simulink model "EcoSIM3_P2_C2"  (R2014b)
settings: Solver=ode1  SolverMode=SingleTasking  StartTime=0.0  StopTime=inf  FixedStep=0.01  RelTol=1e-3
PostLoadFcn:
  | %, if any(exist('dsrtsu_mdlpostloadfcn', 'file') == [2, 3, 6]), try dsrtsu_mdlpostloadfcn('Execute', bdroot); catch fprintf('Error in PostLoadFcn (dsrtsu_mdlpostloadfcn) for model "%s":\n %s\n', bdroot, lasterr); end, end,
InitFcn:
  | tic
  | %Startup_EcoSIM
undefined symbols (not defined in the file or in its folder): canChannel, Controls, DriveCycles, Driver, EM_EFF_MAP, EM_PwrLoss_MAP, EngPwr, EngSpd, EngTrq, Glbl, Plants, Power, Torque, Veh_Dynamics
libraries: canmsglib x100, canlib x87, fl_lib x78, simulink x59, nesl_utility x40, sdl_lib x17, dspsigops x5, dspswit3 x3, dspstat3 x2, commnoisgen2 x1, dspfdesign x1
(part 11 of 15)

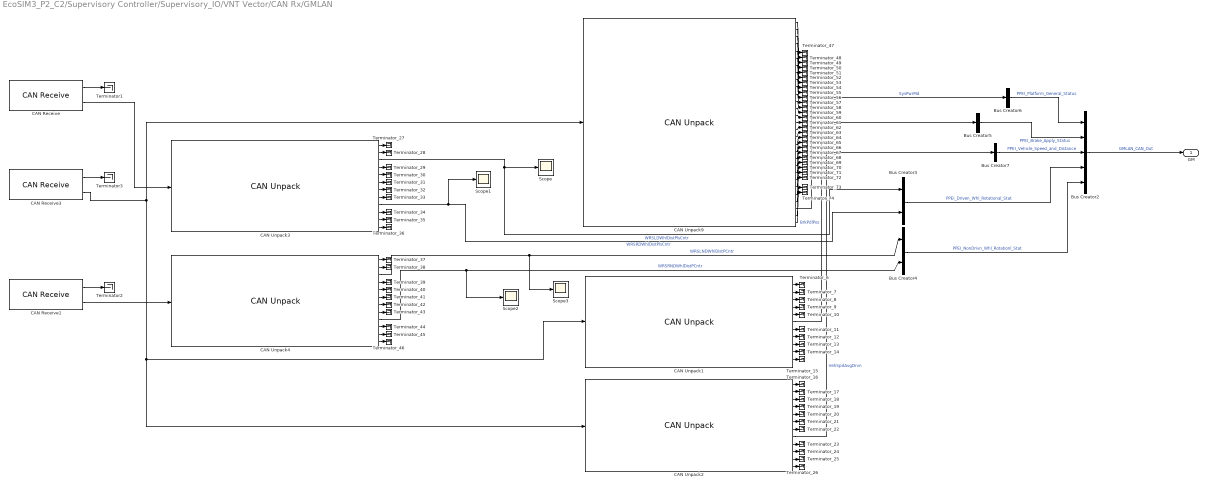
== system EcoSIM3_P2_C2/Supervisory Controller/Supervisory_IO/VNT Vector/CAN Rx/GMLAN ==
  Bus Creator2 : BusCreator  Inputs=5
  Bus Creator3 : BusCreator  Inputs=2
  Bus Creator4 : BusCreator  Inputs=2
  Bus Creator5 : BusCreator  Inputs=1
  Bus Creator6 : BusCreator  Inputs=1
  Bus Creator7 : BusCreator  Inputs=1
  CAN Receive : canlib/CAN Receive  BlockHandle=34350.0007  DeviceMenu=Vector Virtual 1 (Channel 1)  Device=Vector Virtual 1 (Channel 1)  ObjConstructor=canChannel('Vector', 'Virtual 1', 1)  EnableStandardIDsFilter=off  StandardIDs=193  EnableExtendedIDsFilter=off  ExtendedIDs=0  SampleTime=0.01  MsgsPerTimestep=all  StdIDsCombo=Allow only  ExtIDsCombo=Allow all  InternalFilterUpdateStatus=on
  CAN Receive1 : canlib/CAN Receive  BlockHandle=34351.0004  DeviceMenu=Vector Virtual 1 (Channel 1)  Device=Vector Virtual 1 (Channel 1)  ObjConstructor=canChannel('Vector', 'Virtual 1', 1)  EnableStandardIDsFilter=off  StandardIDs=197  EnableExtendedIDsFilter=off  ExtendedIDs=0  SampleTime=0.01  MsgsPerTimestep=all  StdIDsCombo=Allow only  ExtIDsCombo=Allow all  InternalFilterUpdateStatus=on
  CAN Receive3 : canlib/CAN Receive  BlockHandle=34352.0004  DeviceMenu=Vector Virtual 1 (Channel 1)  Device=Vector Virtual 1 (Channel 1)  ObjConstructor=canChannel('Vector', 'Virtual 1', 1)  EnableStandardIDsFilter=off  StandardIDs=[193 197 241 497 1001]  EnableExtendedIDsFilter=off  ExtendedIDs=0  SampleTime=0.01  MsgsPerTimestep=1  StdIDsCombo=Allow only  ExtIDsCombo=Block all  InternalFilterUpdateStatus=on
  CAN Unpack1 : canmsglib/CAN Unpack  CANdbFile=C:\Users\EcoCAR_HIL\Documents\Khanna\EcoSIM3_P1_0_PHEV_TCU\Final_DBC\GlobalAHS_anon GM CONFIDENTIAL.dbc  MsgList=PPEI_Brake_Apply_Status  MsgName=PPEI_Brake_Apply_Status  MsgIDType=Standard (11-bit identifier)  MsgIdentifier=241  MsgLength=6  SignalInfo=BrkAppSnsrHmPosLrnd$30$1$2$2$1$0$1$0$0$1$#BrkPdlChkData$40$17$2$2$1$0$1$0$0$131071$#BrkPdlInTrvPrt$2$2$2$2$1$0$1$0$0$3$#BrkPdlModTrvl$6$1$2$2$1$0$1$0$0$1$#BrkPdlModTrvlV$7$1$2$2$1$0$1$0$0$1$#BrkPdlPos$8$8$2$2$1$0$3.921570e-01$0$0$1.000000e+02$#BrkPdlPosGrad$16$8$2$1$1$0$40$0$-5120$5080$#BrkPedPosAlvRolngCnt$4$2$2$2$1$0$1$0$0$3$#BrkPedTrvlAchvd$1$1$2$2$1$0$1$0$0$1$#BrkPedTrvlAchvdV$0$1$2$2$1$0$1$0$0$1$#NotEventStat$28$2$2$2$1$0$1$0$0$3$#  NSignals=11  IDPort=off  TimestampPort=off  ErrorPort=off  RemotePort=off  LengthPort=off  StatusPort=off  StartBits=str2num('[int32(30);int32(40);int32(2);int32(6);int32(7);int32(8);int32(16);int32(4);int32(1);int32(0);int32(28)]')  SignalSizes=str2num('[int32(1);int32(17);int32(2);int32(1);int32(1);int32(8);int32(8);int32(2);int32(1);int32(1);int32(2)]')  ByteOrders=str2num('[int32(2);int32(2);int32(2);int32(2);int32(2);int32(2);int32(2);int32(2);int32(2);int32(2);int32(2)]')  DataTypes=str2num('[int32(2);int32(2);int32(2);int32(2);int32(2);int32(2);int32(1);int32(2);int32(2);int32(2);int32(2)]')  MultiplexTypes=str2num('[int32(1);int32(1);int32(1);int32(1);int32(1);int32(1);int32(1);int32(1);int32(1);int32(1);int32(1)]')  MultiplexValues=str2num('[double(0);double(0);double(0);double(0);double(0);double(0);double(0);double(0);double(0);double(0);double(0)]')  Factors=str2num('[double(1);double(1);double(1);double(1);double(1);double(3.921570e-01);double(40);double(1);double(1);double(1);double(1)]')  Offsets=str2num('[double(0);double(0);double(0);double(0);double(0);double(0);double(0);double(0);double(0);double(0);double(0)]')  Minimums=str2num('[double(0);double(0);double(0);double(0);double(0);double(0);double(-5120);double(0);double(0);double(0);double(0)]')  Maximums=str2num('[double(1);double(131071);double(3);double(1);double(1);double(1.000000e+02);double(5080);double(3);double(1);double(1);double(3)]')
      settings: DataFormat=CANdb specified signals
  CAN Unpack2 : canmsglib/CAN Unpack  CANdbFile=C:\Users\EcoCAR_HIL\Documents\Khanna\EcoSIM3_P1_0_PHEV_TCU\Final_DBC\GlobalAHS_anon GM CONFIDENTIAL.dbc  MsgList=PPEI_Vehicle_Speed_and_Distance  MsgName=PPEI_Vehicle_Speed_and_Distance  MsgIDType=Standard (11-bit identifier)  MsgIdentifier=1001  MsgLength=8  SignalInfo=DistRollCntAvgDrvn$24$13$2$2$1$0$1.250000e-01$0$0$1.023875e+03$#DistRollCntAvgDrvnSrc$55$1$2$2$1$0$1$0$0$1$#DistRollCntAvgDrvnV$22$1$2$2$1$0$1$0$0$1$#DstRolCntAvNDrRstOc$53$1$2$2$1$0$1$0$0$1$#DstRolCntAvgDrnRstOc$21$1$2$2$1$0$1$0$0$1$#DstRolCntAvgNonDrvn$56$13$2$2$1$0$1.250000e-01$0$0$1.023875e+03$#DstRolCntAvgNonDrvnV$54$1$2$2$1$0$1$0$0$1$#VehSpdAvgDrvn$8$15$2$2$1$0$1.562500e-02$0$0$5.119844e+02$#VehSpdAvgDrvnSrc$23$1$2$2$1$0$1$0$0$1$#VehSpdAvgDrvnV$7$1$2$2$1$0$1$0$0$1$#VehSpdAvgNDrvn$40$15$2$2$1$0$1.562500e-02$0$0$5.119844e+02$#VehSpdAvgNDrvnV$39$1$2$2$1$0$1$0$0$1$#  NSignals=12  IDPort=off  TimestampPort=off  ErrorPort=off  RemotePort=off  LengthPort=off  StatusPort=off  StartBits=str2num('[int32(24);int32(55);int32(22);int32(53);int32(21);int32(56);int32(54);int32(8);int32(23);int32(7);int32(40);int32(39)]')  SignalSizes=str2num('[int32(13);int32(1);int32(1);int32(1);int32(1);int32(13);int32(1);int32(15);int32(1);int32(1);int32(15);int32(1)]')  ByteOrders=str2num('[int32(2);int32(2);int32(2);int32(2);int32(2);int32(2);int32(2);int32(2);int32(2);int32(2);int32(2);int32(2)]')  DataTypes=str2num('[int32(2);int32(2);int32(2);int32(2);int32(2);int32(2);int32(2);int32(2);int32(2);int32(2);int32(2);int32(2)]')  MultiplexTypes=str2num('[int32(1);int32(1);int32(1);int32(1);int32(1);int32(1);int32(1);int32(1);int32(1);int32(1);int32(1);int32(1)]')  MultiplexValues=str2num('[double(0);double(0);double(0);double(0);double(0);double(0);double(0);double(0);double(0);double(0);double(0);double(0)]')  Factors=str2num('[double(1.250000e-01);double(1);double(1);double(1);double(1);double(1.250000e-01);double(1);double(1.562500e-02);double(1);double(1);double(1.562500e-02);double(1)]')  Offsets=str2num('[double(0);double(0);double(0);double(0);double(0);double(0);double(0);double(0);double(0);double(0);double(0);double(0)]')  Minimums=str2num('[double(0);double(0);double(0);double(0);double(0);double(0);double(0);double(0);double(0);double(0);double(0);double(0)]')  Maximums=str2num('[double(1.023875e+03);double(1);double(1);double(1);double(1);double(1.023875e+03);double(1);double(5.119844e+02);double(1);double(1);double(5.119844e+02);double(1)]')
      settings: DataFormat=CANdb specified signals
  CAN Unpack3 : canmsglib/CAN Unpack  CANdbFile=C:\Users\EcoCAR_HIL\Documents\Khanna\EcoSIM3_P1_0_PHEV_TCU\Final_DBC\GlobalAHS_anon GM CONFIDENTIAL.dbc  MsgList=PPEI_Driven_Whl_Rotational_Stat  MsgName=PPEI_Driven_Whl_Rotational_Stat  MsgIDType=Standard (11-bit identifier)  MsgIdentifier=193  MsgLength=8  SignalInfo=WRSLDSeqNum$4$2$2$2$1$0$1$0$0$3$#WRSLDWhlDisTpRC$6$2$2$2$1$0$1$0$0$3$#WRSLDWhlDistPlsCntr$8$10$2$2$1$0$1$0$0$1023$#WRSLDWhlDistTmstm$24$16$2$2$1$0$1$0$0$65535$#WRSLDWhlDistVal$2$1$2$2$1$0$1$0$0$1$#WRSLDWhlRotStatRst$3$1$2$2$1$0$1$0$0$1$#WRSRDSeqNum$36$2$2$2$1$0$1$0$0$3$#WRSRDWhlDisTpRC$38$2$2$2$1$0$1$0$0$3$#WRSRDWhlDistPlsCntr$40$10$2$2$1$0$1$0$0$1023$#WRSRDWhlDistTmstm$56$16$2$2$1$0$1$0$0$65535$#WRSRDWhlDistVal$34$1$2$2$1$0$1$0$0$1$#WRSRDWhlRotStatRst$35$1$2$2$1$0$1$0$0$1$#  NSignals=12  IDPort=off  TimestampPort=off  ErrorPort=off  RemotePort=off  LengthPort=off  StatusPort=off  StartBits=str2num('[int32(4);int32(6);int32(8);int32(24);int32(2);int32(3);int32(36);int32(38);int32(40);int32(56);int32(34);int32(35)]')  SignalSizes=str2num('[int32(2);int32(2);int32(10);int32(16);int32(1);int32(1);int32(2);int32(2);int32(10);int32(16);int32(1);int32(1)]')  ByteOrders=str2num('[int32(2);int32(2);int32(2);int32(2);int32(2);int32(2);int32(2);int32(2);int32(2);int32(2);int32(2);int32(2)]')  DataTypes=str2num('[int32(2);int32(2);int32(2);int32(2);int32(2);int32(2);int32(2);int32(2);int32(2);int32(2);int32(2);int32(2)]')  MultiplexTypes=str2num('[int32(1);int32(1);int32(1);int32(1);int32(1);int32(1);int32(1);int32(1);int32(1);int32(1);int32(1);int32(1)]')  MultiplexValues=str2num('[double(0);double(0);double(0);double(0);double(0);double(0);double(0);double(0);double(0);double(0);double(0);double(0)]')  Factors=str2num('[double(1);double(1);double(1);double(1);double(1);double(1);double(1);double(1);double(1);double(1);double(1);double(1)]')  Offsets=str2num('[double(0);double(0);double(0);double(0);double(0);double(0);double(0);double(0);double(0);double(0);double(0);double(0)]')  Minimums=str2num('[double(0);double(0);double(0);double(0);double(0);double(0);double(0);double(0);double(0);double(0);double(0);double(0)]')  Maximums=str2num('[double(3);double(3);double(1023);double(65535);double(1);double(1);double(3);double(3);double(1023);double(65535);double(1);double(1)]')
      settings: DataFormat=CANdb specified signals
  CAN Unpack4 : canmsglib/CAN Unpack  CANdbFile=C:\Users\EcoCAR_HIL\Documents\Khanna\EcoSIM3_P1_0_PHEV_TCU\Final_DBC\GlobalAHS_anon GM CONFIDENTIAL.dbc  MsgList=PPEI_NonDrivn_Whl_Rotationl_Stat  MsgName=PPEI_NonDrivn_Whl_Rotationl_Stat  MsgIDType=Standard (11-bit identifier)  MsgIdentifier=197  MsgLength=8  SignalInfo=WRSLNDSeqNum$4$2$2$2$1$0$1$0$0$3$#WRSLNDWhlDisTpRC$6$2$2$2$1$0$1$0$0$3$#WRSLNDWhlDistPCntr$8$10$2$2$1$0$1$0$0$1023$#WRSLNDWhlDistTstm$24$16$2$2$1$0$1$0$0$65535$#WRSLNDWhlDistVal$2$1$2$2$1$0$1$0$0$1$#WRSLNDWhlRotStRst$3$1$2$2$1$0$1$0$0$1$#WRSRNDSeqNum$36$2$2$2$1$0$1$0$0$3$#WRSRNDWhlDisTpRC$38$2$2$2$1$0$1$0$0$3$#WRSRNDWhlDistPCntr$40$10$2$2$1$0$1$0$0$1023$#WRSRNDWhlDistTstm$56$16$2$2$1$0$1$0$0$65535$#WRSRNDWhlDistVal$34$1$2$2$1$0$1$0$0$1$#WRSRNDWhlRotStRst$35$1$2$2$1$0$1$0$0$1$#  NSignals=12  IDPort=off  TimestampPort=off  ErrorPort=off  RemotePort=off  LengthPort=off  StatusPort=off  StartBits=str2num('[int32(4);int32(6);int32(8);int32(24);int32(2);int32(3);int32(36);int32(38);int32(40);int32(56);int32(34);int32(35)]')  SignalSizes=str2num('[int32(2);int32(2);int32(10);int32(16);int32(1);int32(1);int32(2);int32(2);int32(10);int32(16);int32(1);int32(1)]')  ByteOrders=str2num('[int32(2);int32(2);int32(2);int32(2);int32(2);int32(2);int32(2);int32(2);int32(2);int32(2);int32(2);int32(2)]')  DataTypes=str2num('[int32(2);int32(2);int32(2);int32(2);int32(2);int32(2);int32(2);int32(2);int32(2);int32(2);int32(2);int32(2)]')  MultiplexTypes=str2num('[int32(1);int32(1);int32(1);int32(1);int32(1);int32(1);int32(1);int32(1);int32(1);int32(1);int32(1);int32(1)]')  MultiplexValues=str2num('[double(0);double(0);double(0);double(0);double(0);double(0);double(0);double(0);double(0);double(0);double(0);double(0)]')  Factors=str2num('[double(1);double(1);double(1);double(1);double(1);double(1);double(1);double(1);double(1);double(1);double(1);double(1)]')  Offsets=str2num('[double(0);double(0);double(0);double(0);double(0);double(0);double(0);double(0);double(0);double(0);double(0);double(0)]')  Minimums=str2num('[double(0);double(0);double(0);double(0);double(0);double(0);double(0);double(0);double(0);double(0);double(0);double(0)]')  Maximums=str2num('[double(3);double(3);double(1023);double(65535);double(1);double(1);double(3);double(3);double(1023);double(65535);double(1);double(1)]')
      settings: DataFormat=CANdb specified signals
  CAN Unpack9 : canmsglib/CAN Unpack  CANdbFile=C:\Users\EcoCAR_HIL\Documents\Khanna\EcoSIM3_P1_0_PHEV_TCU\Final_DBC\GlobalAHS_anon GM CONFIDENTIAL.dbc  MsgList=PPEI_Platform_General_Status  MsgName=PPEI_Platform_General_Status  MsgIDType=Standard (11-bit identifier)  MsgIdentifier=497  MsgLength=8  SignalInfo=ACCmpsrFldOn$63$1$2$2$1$0$1$0$0$1$#ACCompModReq$11$2$2$2$1$0$1$0$0$3$#ACCompNormLd$48$8$2$2$1$0$1.000000e-01$0$0$2.550000e+01$#ACCompNormLdV$10$1$2$2$1$0$1$0$0$1$#ACCompSysVDA$9$1$2$2$1$0$1$0$0$1$#ACCompSysVDM$60$1$2$2$1$0$1$0$0$1$#AirbgVDA$57$1$2$2$1$0$1$0$0$1$#BkupPwrModeMstrVDA$7$1$2$2$1$0$1$0$0$1$#BkupPwrModeMstrVDM$61$1$2$2$1$0$1$0$0$1$#DispMeasSys$59$1$2$2$1$0$1$0$0$1$#ElvtdIdlCstStReq$32$2$2$2$1$0$1$0$0$3$#EngOilLfRstRq$37$1$2$2$1$0$1$0$0$1$#FuelFltLfRstRqd$56$1$2$2$1$0$1$0$0$1$#ImmblzrPreRelPswdStat$8$1$2$2$1$0$1$0$0$1$#ImmblzrPreRelPswrd$24$16$2$2$1$0$1$0$0$65535$#PMMAccTrmSt$2$1$2$2$1$0$1$0$0$1$#PMMRunCrkTrmSt$3$1$2$2$1$0$1$0$0$1$#PTORSMstrEngShtReq$13$1$2$2$1$0$1$0$0$1$#PTORmStMsEngStRq$14$1$2$2$1$0$1$0$0$1$#PrkBrkSwAtv$36$1$2$2$1$0$1$0$0$1$#PrkBrkVDA$35$1$2$2$1$0$1$0$0$1$#PrkBrkVDM$62$1$2$2$1$0$1$0$0$1$#RmVehStrRq$15$1$2$2$1$0$1$0$0$1$#SIRDpl$58$1$2$2$1$0$1$0$0$1$#SysBkUpPwrMd$4$2$2$2$1$0$1$0$0$3$#SysBkupPwrMdEn$6$1$2$2$1$0$1$0$0$1$#SysPwrMd$0$2$2$2$1$0$1$0$0$3$#ThrtlPrgrsnReq$38$2$2$2$1$0$1$0$0$3$#TrStLgMdAtv$34$1$2$2$1$0$1$0$0$1$#  NSignals=29  IDPort=off  TimestampPort=off  ErrorPort=off  RemotePort=off  LengthPort=off  StatusPort=off  StartBits=str2num('[int32(63);int32(11);int32(48);int32(10);int32(9);int32(60);int32(57);int32(7);int32(61);int32(59);int32(32);int32(37);int32(56);int32(8);int32(24);int32(2);int32(3);int32(13);int32(14);int32(36);int32(35);int32(62);int32(15);int32(58);int32(4);int32(6);int32(0);int32(38);int32(34)]')  SignalSizes=str2num('[int32(1);int32(2);int32(8);int32(1);int32(1);int32(1);int32(1);int32(1);int32(1);int32(1);int32(2);int32(1);int32(1);int32(1);int32(16);int32(1);int32(1);int32(1);int32(1);int32(1);int32(1);int32(1);int32(1);int32(1);int32(2);int32(1);int32(2);int32(2);int32(1)]')  ByteOrders=str2num('[int32(2);int32(2);int32(2);int32(2);int32(2);int32(2);int32(2);int32(2);int32(2);int32(2);int32(2);int32(2);int32(2);int32(2);int32(2);int32(2);int32(2);int32(2);int32(2);int32(2);int32(2);int32(2);int32(2);int32(2);int32(2);int32(2);int32(2);int32(2);int32(2)]')  DataTypes=str2num('[int32(2);int32(2);int32(2);int32(2);int32(2);int32(2);int32(2);int32(2);int32(2);int32(2);int32(2);int32(2);int32(2);int32(2);int32(2);int32(2);int32(2);int32(2);int32(2);int32(2);int32(2);int32(2);int32(2);int32(2);int32(2);int32(2);int32(2);int32(2);int32(2)]')  MultiplexTypes=str2num('[int32(1);int32(1);int32(1);int32(1);int32(1);int32(1);int32(1);int32(1);int32(1);int32(1);int32(1);int32(1);int32(1);int32(1);int32(1);int32(1);int32(1);int32(1);int32(1);int32(1);int32(1);int32(1);int32(1);int32(1);int32(1);int32(1);int32(1);int32(1);int32(1)]')  MultiplexValues=str2num('[double(0);double(0);double(0);double(0);double(0);double(0);double(0);double(0);double(0);double(0);double(0);double(0);double(0);double(0);double(0);double(0);double(0);double(0);double(0);double(0);double(0);double(0);double(0);double(0);double(0);double(0);double(0);double(0);double(0)]')  Factors=str2num('[double(1);double(1);double(1.000000e-01);double(1);double(1);double(1);double(1);double(1);double(1);double(1);double(1);double(1);double(1);double(1);double(1);double(1);double(1);double(1);double(1);double(1);double(1);double(1);double(1);double(1);double(1);double(1);double(1);double(1);double(1)]')  Offsets=str2num('[double(0);double(0);double(0);double(0);double(0);double(0);double(0);double(0);double(0);double(0);double(0);double(0);double(0);double(0);double(0);double(0);double(0);double(0);double(0);double(0);double(0);double(0);double(0);double(0);double(0);double(0);double(0);double(0);double(0)]')  Minimums=str2num('[double(0);double(0);double(0);double(0);double(0);double(0);double(0);double(0);double(0);double(0);double(0);double(0);double(0);double(0);double(0);double(0);double(0);double(0);double(0);double(0);double(0);double(0);double(0);double(0);double(0);double(0);double(0);double(0);double(0)]')  Maximums=str2num('[double(1);double(3);double(2.550000e+01);double(1);double(1);double(1);double(1);double(1);double(1);double(1);double(3);double(1);double(1);double(1);double(65535);double(1);double(1);double(1);double(1);double(1);double(1);double(1);double(1);double(1);double(3);double(1);double(3);double(3);double(1)]')
      settings: DataFormat=CANdb specified signals
  Scope{,1..3} (4 alike) : Scope
      Scope settings: TimeRange=20  YMin=0  YMax=3  SaveName=ScopeData19
      Scope1 settings: TimeRange=20  YMin=0  YMax=3  SaveName=ScopeData5
      Scope2 settings: TimeRange=20  YMin=0  YMax=3  SaveName=ScopeData15
      Scope3 settings: TimeRange=20  YMin=0  YMax=3  SaveName=ScopeData24
  Terminator1 : Terminator
  Terminator2 : Terminator
  Terminator3 : Terminator
  Terminator_{6..74} (69 alike) : Terminator
  GM : Outport
  wires:
  CAN Unpack4/3 -> Scope3/1, Bus Creator4/1  "WRSLNDWhlDistPCntr"
  CAN Unpack3/3 -> Bus Creator3/1, Scope/1  "WRSLDWhlDistPlsCntr"
  Bus Creator4/1 -> Bus Creator2/5  "PPEI_NonDrivn_Whl_Rotationl_Stat"
  Bus Creator3/1 -> Bus Creator2/4  "PPEI_Driven_Whl_Rotational_Stat"
  CAN Unpack4/9 -> Scope2/1, Bus Creator4/2  "WRSRNDWhlDistPCntr"
  CAN Unpack3/9 -> Scope1/1, Bus Creator3/2  "WRSRDWhlDistPlsCntr"
  Bus Creator2/1 -> GM/1  "GMLAN_CAN_Out"
  Bus Creator5/1 -> Bus Creator2/2  "PPEI_Brake_Apply_Status"
  Bus Creator6/1 -> Bus Creator2/1  "PPEI_Platform_General_Status"
  CAN Unpack2/8 -> Bus Creator7/1  "VehSpdAvgDrvn"
  Bus Creator7/1 -> Bus Creator2/3  "PPEI_Vehicle_Speed_and_Distance"
  CAN Unpack1/6 -> Bus Creator5/1  "BrkPdlPos"
  CAN Unpack9/27 -> Bus Creator6/1  "SysPwrMd"
  CAN Receive3/2 -> CAN Unpack9/1, CAN Unpack2/1, CAN Unpack1/1
  CAN Receive3/1 -> Terminator3/1
  CAN Unpack1/1 -> Terminator_6/1
  CAN Unpack1/2 -> Terminator_7/1
  CAN Unpack1/3 -> Terminator_8/1
  CAN Unpack1/4 -> Terminator_9/1
  CAN Unpack1/5 -> Terminator_10/1
  CAN Unpack1/7 -> Terminator_11/1
  CAN Unpack1/8 -> Terminator_12/1
  CAN Unpack1/9 -> Terminator_13/1
  CAN Unpack1/10 -> Terminator_14/1
  CAN Unpack1/11 -> Terminator_15/1
  CAN Unpack2/1 -> Terminator_16/1
  CAN Unpack2/2 -> Terminator_17/1
  CAN Unpack2/3 -> Terminator_18/1
  CAN Unpack2/4 -> Terminator_19/1
  CAN Unpack2/5 -> Terminator_20/1
  CAN Unpack2/6 -> Terminator_21/1
  CAN Unpack2/7 -> Terminator_22/1
  CAN Unpack2/9 -> Terminator_23/1
  CAN Unpack2/10 -> Terminator_24/1
  CAN Unpack2/11 -> Terminator_25/1
  CAN Unpack2/12 -> Terminator_26/1
  CAN Unpack3/1 -> Terminator_27/1
  CAN Unpack3/2 -> Terminator_28/1
  CAN Unpack3/4 -> Terminator_29/1
  CAN Unpack3/5 -> Terminator_30/1
  CAN Unpack3/6 -> Terminator_31/1
  CAN Unpack3/7 -> Terminator_32/1
  CAN Unpack3/8 -> Terminator_33/1
  CAN Unpack3/10 -> Terminator_34/1
  CAN Unpack3/11 -> Terminator_35/1
  CAN Unpack3/12 -> Terminator_36/1
  CAN Unpack4/1 -> Terminator_37/1
  CAN Unpack4/2 -> Terminator_38/1
  CAN Unpack4/4 -> Terminator_39/1
  CAN Unpack4/5 -> Terminator_40/1
  CAN Unpack4/6 -> Terminator_41/1
  CAN Unpack4/7 -> Terminator_42/1
  CAN Unpack4/8 -> Terminator_43/1
  CAN Unpack4/10 -> Terminator_44/1
  CAN Unpack4/11 -> Terminator_45/1
  CAN Unpack4/12 -> Terminator_46/1
  CAN Unpack9/1 -> Terminator_47/1
  CAN Unpack9/2 -> Terminator_48/1
  CAN Unpack9/3 -> Terminator_49/1
  CAN Unpack9/4 -> Terminator_50/1
  CAN Unpack9/5 -> Terminator_51/1
  CAN Unpack9/6 -> Terminator_52/1
  CAN Unpack9/7 -> Terminator_53/1
  CAN Unpack9/8 -> Terminator_54/1
  CAN Unpack9/9 -> Terminator_55/1
  CAN Unpack9/10 -> Terminator_56/1
  CAN Unpack9/11 -> Terminator_57/1
  CAN Unpack9/12 -> Terminator_58/1
  CAN Unpack9/13 -> Terminator_59/1
  CAN Unpack9/14 -> Terminator_60/1
  CAN Unpack9/15 -> Terminator_61/1
  CAN Unpack9/16 -> Terminator_62/1
  CAN Unpack9/17 -> Terminator_63/1
  CAN Unpack9/18 -> Terminator_64/1
  CAN Unpack9/19 -> Terminator_65/1
  CAN Unpack9/20 -> Terminator_66/1
  CAN Unpack9/21 -> Terminator_67/1
  CAN Unpack9/22 -> Terminator_68/1
  CAN Unpack9/23 -> Terminator_69/1
  CAN Unpack9/24 -> Terminator_70/1
  CAN Unpack9/25 -> Terminator_71/1
  CAN Unpack9/26 -> Terminator_72/1
  CAN Unpack9/28 -> Terminator_73/1
  CAN Unpack9/29 -> Terminator_74/1
  CAN Receive/1 -> Terminator1/1
  CAN Receive/2 -> CAN Unpack3/1
  CAN Receive1/2 -> CAN Unpack4/1
  CAN Receive1/1 -> Terminator2/1

== system EcoSIM3_P2_C2/Supervisory Controller/Supervisory_IO/VNT Vector/CAN Tx/ESS ==
  ESS : Inport
  Bus Selector2 : BusSelector  OutputSignals=ESS_Signals_A123.hsc_bcm_enable,ESS_Signals_A123.hsc_bcm_epo,ESS_Signals_A123.hsc_bcm_leakage_ena,ESS_Signals_A123.hsc_bcm_mainc_close
  CAN Pack4 : canmsglib/CAN Pack  CANdbFile=C:\Users\EcoCAR_HIL\Documents\Khanna\EcoSIM3_P1_0_PHEV_TCU\Final_DBC\BCM_VehBus_Std.dbc  MsgList=BCM_Request  MsgName=BCM_Request  MsgIDType=Standard (11-bit identifier)  MsgIdentifier=1024  MsgLength=4  SignalInfo=hsc_bcm_enable$0$1$2$2$1$0$1$0$0$1$#hsc_bcm_epo$1$1$2$2$1$0$1$0$0$1$#hsc_bcm_leakage_ena$3$1$2$2$1$0$1$0$0$1$#hsc_bcm_mainc_close$2$1$2$2$1$0$1$0$0$1$#  NSignals=4  StartBits=str2num('[int32(0);int32(1);int32(3);int32(2)]')  SignalSizes=str2num('[int32(1);int32(1);int32(1);int32(1)]')  ByteOrders=str2num('[int32(2);int32(2);int32(2);int32(2)]')  DataTypes=str2num('[int32(2);int32(2);int32(2);int32(2)]')  MultiplexTypes=str2num('[int32(1);int32(1);int32(1);int32(1)]')  MultiplexValues=str2num('[double(0);double(0);double(0);double(0)]')  Factors=str2num('[double(1);double(1);double(1);double(1)]')  Offsets=str2num('[double(0);double(0);double(0);double(0)]')  Minimums=str2num('[double(0);double(0);double(0);double(0)]')  Maximums=str2num('[double(1);double(1);double(1);double(1)]')  Remote=off
      settings: DataFormat=CANdb specified signals
  CAN Transmit4 : canlib/CAN Transmit  BlockHandle=13189.0195  DeviceMenu=Vector Virtual 1 (Channel 1)  Device=Vector Virtual 1 (Channel 1)  ObjConstructor=canChannel('Vector', 'Virtual 1', 1)  EnablePeriodicTransmit=off  MessagePeriod=1.000
  Rate Transition{,1..3} (4 alike) : RateTransition
  wires:
  ESS/1 -> Bus Selector2/1
  Bus Selector2/2 -> Rate Transition1/1  "<hsc_bcm_epo>"
  Bus Selector2/3 -> Rate Transition2/1  "<hsc_bcm_leakage_ena>"
  CAN Pack4/1 -> CAN Transmit4/1
  Bus Selector2/4 -> Rate Transition3/1  "<hsc_bcm_mainc_close>"
  Bus Selector2/1 -> Rate Transition/1  "<hsc_bcm_enable>"
  Rate Transition/1 -> CAN Pack4/1
  Rate Transition1/1 -> CAN Pack4/2
  Rate Transition2/1 -> CAN Pack4/3
  Rate Transition3/1 -> CAN Pack4/4

== system EcoSIM3_P2_C2/Supervisory Controller/Supervisory_IO/VNT Vector/CAN Tx/Eelctric Motor ==
  EMTransmit : Inport
  Bus Selector : BusSelector  OutputSignals=Rotation_Direction,Inverter_Enable,Torque_Command
  Bus Selector1 : BusSelector  OutputSignals=EM_Messages_Rhinehart
  CAN Pack : canmsglib/CAN Pack  CANdbFile=C:\Users\EcoCAR_HIL\Documents\Khanna\EcoSIM3_P1_0_PHEV_TCU\Final_DBC\20160113 RMS PM CAN DB.dbc  MsgList=M192_Command_Message  MsgName=M192_Command_Message  MsgIDType=Standard (11-bit identifier)  MsgIdentifier=192  MsgLength=8  SignalInfo=Direction_Command$32$1$1$2$1$0$1$0$0$1$#Inverter_Discharge$41$1$1$2$1$0$1$0$0$1$#Inverter_Enable$40$1$1$2$1$0$1$0$0$1$#Speed_Command$16$16$1$1$1$0$1$0$-32768$32767$#Speed_Mode_Enable$42$1$1$2$1$0$1$0$0$1$#Torque_Command$0$16$1$1$1$0$1.000000e-01$0$-3.276800e+03$3.276700e+03$#Torque_Limit_Command$48$16$1$1$1$0$1$0$-3.276800e+03$3.276700e+03$#  NSignals=7  StartBits=str2num('[int32(32);int32(41);int32(40);int32(16);int32(42);int32(0);int32(48)]')  SignalSizes=str2num('[int32(1);int32(1);int32(1);int32(16);int32(1);int32(16);int32(16)]')  ByteOrders=str2num('[int32(1);int32(1);int32(1);int32(1);int32(1);int32(1);int32(1)]')  DataTypes=str2num('[int32(2);int32(2);int32(2);int32(1);int32(2);int32(1);int32(1)]')  MultiplexTypes=str2num('[int32(1);int32(1);int32(1);int32(1);int32(1);int32(1);int32(1)]')  MultiplexValues=str2num('[double(0);double(0);double(0);double(0);double(0);double(0);double(0)]')  Factors=str2num('[double(1);double(1);double(1);double(1);double(1);double(1.000000e-01);double(1)]')  Offsets=str2num('[double(0);double(0);double(0);double(0);double(0);double(0);double(0)]')  Minimums=str2num('[double(0);double(0);double(0);double(-32768);double(0);double(-3.276800e+03);double(-3.276800e+03)]')  Maximums=str2num('[double(1);double(1);double(1);double(32767);double(1);double(3.276700e+03);double(3.276700e+03)]')  Remote=off
      settings: DataFormat=CANdb specified signals
  CAN Transmit : canlib/CAN Transmit  BlockHandle=13209.0195  DeviceMenu=Vector Virtual 1 (Channel 1)  Device=Vector Virtual 1 (Channel 2)  ObjConstructor=canChannel('Vector', 'Virtual 1', 2)  EnablePeriodicTransmit=off  MessagePeriod=1.000
  Ground_{1..4} (4 alike) : Ground
  Rate Transition : RateTransition
  Rate Transition1 : RateTransition
  Rate Transition2 : RateTransition
  wires:
  EMTransmit/1 -> Bus Selector1/1
  Bus Selector/2 -> Rate Transition1/1  "<Inverter_Enable>"
  Bus Selector/3 -> Rate Transition2/1  "<Torque_Command>"
  Bus Selector/1 -> Rate Transition/1  "<Rotation_Direction>"
  CAN Pack/1 -> CAN Transmit/1
  Bus Selector1/1 -> Bus Selector/1  "<EM_Messages_Rhinehart>"
  Rate Transition/1 -> CAN Pack/1
  Rate Transition1/1 -> CAN Pack/3
  Rate Transition2/1 -> CAN Pack/6
  Ground_1/1 -> CAN Pack/2
  Ground_2/1 -> CAN Pack/4
  Ground_3/1 -> CAN Pack/5
  Ground_4/1 -> CAN Pack/7

== system EcoSIM3_P2_C2/Supervisory Controller/Supervisory_IO/VNT Vector/CAN Tx/ICE_BAS_Trans ==
  ICE_BAS_Trans : Inport
  Bus Selector1 : BusSelector  OutputSignals=Engine_Messages.ICE_Torque_Request_Nm,Engine_Messages.Engine_Run,Engine_Messages.Engine_On,BAS_SoftECU_Receive.BAS_Mode_Request,BAS_SoftECU_Receive.BAS_Torque_Request_Nm,Trans_Receive.Gear_Request
  CAN Pack1 : canmsglib/CAN Pack  CANdbFile=C:\Users\EcoCAR_HIL\Box Sync\EcoCAR 3\SMS\EcoSIM3_P2_C2\MIL\Final_DBC\Engine_Transmission_BAS.dbc  MsgList=ECO_Engine_MSG101  MsgName=ECO_Engine_MSG101  MsgIDType=Standard (11-bit identifier)  MsgIdentifier=101  MsgLength=3  SignalInfo=ICE_Torque_Request_Nm$9$15$2$2$1$0$1.000000e-02$0$0$3.276700e+02$#ISP_R$8$1$2$2$1$0$1$0$0$1$#PCM_Wake$23$1$2$2$1$0$1$0$0$1$#  NSignals=3  StartBits=str2num('[int32(9);int32(8);int32(23)]')  SignalSizes=str2num('[int32(15);int32(1);int32(1)]')  ByteOrders=str2num('[int32(2);int32(2);int32(2)]')  DataTypes=str2num('[int32(2);int32(2);int32(2)]')  MultiplexTypes=str2num('[int32(1);int32(1);int32(1)]')  MultiplexValues=str2num('[double(0);double(0);double(0)]')  Factors=str2num('[double(1.000000e-02);double(1);double(1)]')  Offsets=str2num('[double(0);double(0);double(0)]')  Minimums=str2num('[double(0);double(0);double(0)]')  Maximums=str2num('[double(3.276700e+02);double(1);double(1)]')  Remote=off
      settings: DataFormat=CANdb specified signals
  CAN Pack2 : canmsglib/CAN Pack  CANdbFile=C:\Users\EcoCAR_HIL\Documents\Khanna\EcoSIM3_P1_0_PHEV_TCU\Final_DBC\Engine_Transmission_BAS.dbc  MsgList=ECO_BAS_Receive_MSG102  MsgName=ECO_BAS_Receive_MSG102  MsgIDType=Standard (11-bit identifier)  MsgIdentifier=102  MsgLength=2  SignalInfo=BAS_Mode_Request$8$1$2$2$1$0$1$0$0$1$#BAS_Torque_Request_Nm$9$15$2$1$1$0$1.000000e-02$0$-1.638400e+02$1.638300e+02$#  NSignals=2  StartBits=str2num('[int32(8);int32(9)]')  SignalSizes=str2num('[int32(1);int32(15)]')  ByteOrders=str2num('[int32(2);int32(2)]')  DataTypes=str2num('[int32(2);int32(1)]')  MultiplexTypes=str2num('[int32(1);int32(1)]')  MultiplexValues=str2num('[double(0);double(0)]')  Factors=str2num('[double(1);double(1.000000e-02)]')  Offsets=str2num('[double(0);double(0)]')  Minimums=str2num('[double(0);double(-1.638400e+02)]')  Maximums=str2num('[double(1);double(1.638300e+02)]')  Remote=off
      settings: DataFormat=CANdb specified signals
  CAN Pack3 : canmsglib/CAN Pack  CANdbFile=C:\Users\EcoCAR_HIL\Documents\Khanna\EcoSIM3_P1_0_PHEV_TCU\Final_DBC\Engine_Transmission_BAS.dbc  MsgList=ECO_Trans_Receive_MSG105  MsgName=ECO_Trans_Receive_MSG105  MsgIDType=Standard (11-bit identifier)  MsgIdentifier=105  MsgLength=1  SignalInfo=Clutch_Request$4$1$2$2$1$0$1$0$0$1$#Gear_Request$5$3$2$2$1$0$1$0$0$7$#  NSignals=2  StartBits=str2num('[int32(4);int32(5)]')  SignalSizes=str2num('[int32(1);int32(3)]')  ByteOrders=str2num('[int32(2);int32(2)]')  DataTypes=str2num('[int32(2);int32(2)]')  MultiplexTypes=str2num('[int32(1);int32(1)]')  MultiplexValues=str2num('[double(0);double(0)]')  Factors=str2num('[double(1);double(1)]')  Offsets=str2num('[double(0);double(0)]')  Minimums=str2num('[double(0);double(0)]')  Maximums=str2num('[double(1);double(7)]')  Remote=off
      settings: DataFormat=CANdb specified signals
  CAN Transmit1 : canlib/CAN Transmit  BlockHandle=13236.0195  DeviceMenu=(none)  Device=Vector Virtual 1 (Channel 1)  ObjConstructor=canChannel('Vector', 'Virtual 1', 1)  EnablePeriodicTransmit=off  MessagePeriod=1.000
  CAN Transmit2 : canlib/CAN Transmit  BlockHandle=13237.0195  DeviceMenu=(none)  Device=Vector Virtual 1 (Channel 1)  ObjConstructor=canChannel('Vector', 'Virtual 1', 1)  EnablePeriodicTransmit=off  MessagePeriod=1.000
  CAN Transmit3 : canlib/CAN Transmit  BlockHandle=13238.0195  DeviceMenu=Vector Virtual 1 (Channel 1)  Device=Vector Virtual 1 (Channel 1)  ObjConstructor=canChannel('Vector', 'Virtual 1', 1)  EnablePeriodicTransmit=off  MessagePeriod=1.000
  Ground1 : Ground
  Rate Transition{,1..5} (6 alike) : RateTransition
  wires:
  ICE_BAS_Trans/1 -> Bus Selector1/1
  Ground1/1 -> CAN Pack3/1
  CAN Pack2/1 -> CAN Transmit2/1
  Bus Selector1/5 -> Rate Transition2/1  "<BAS_Torque_Request_Nm>"
  Bus Selector1/4 -> Rate Transition1/1  "<BAS_Mode_Request>"
  CAN Pack3/1 -> CAN Transmit3/1
  Bus Selector1/6 -> Rate Transition3/1  "<Gear_Request>"
  CAN Pack1/1 -> CAN Transmit1/1
  Bus Selector1/1 -> Rate Transition/1  "<ICE_Torque_Request_Nm>"
  Rate Transition/1 -> CAN Pack1/1
  Rate Transition1/1 -> CAN Pack2/1
  Rate Transition2/1 -> CAN Pack2/2
  Rate Transition3/1 -> CAN Pack3/2
  Bus Selector1/2 -> Rate Transition4/1  "<Engine_Run>"
  Bus Selector1/3 -> Rate Transition5/1  "<Engine_On>"
  Rate Transition4/1 -> CAN Pack1/2
  Rate Transition5/1 -> CAN Pack1/3

== system EcoSIM3_P2_C2/Supervisory Controller/Supervisory_IO/VNT Vector/CAN Tx/Mode ==
  Mode : Inport
  Bus Selector3 : BusSelector  OutputSignals=Supervisory.Mode
  CAN Pack5 : canmsglib/CAN Pack  CANdbFile=C:\Users\EcoCAR_HIL\Documents\Khanna\EcoSIM3_P1_0_PHEV_TCU\Final_DBC\EcoCAR3_Controls_Development.dbc  MsgList=MABx_Transmit_MSG094  MsgName=MABx_Transmit_MSG094  MsgIDType=Standard (11-bit identifier)  MsgIdentifier=94  MsgLength=1  SignalInfo=Mode$7$1$2$2$1$0$1$0$0$1$#  NSignals=1  StartBits=str2num('[int32(7)]')  SignalSizes=str2num('[int32(1)]')  ByteOrders=str2num('[int32(2)]')  DataTypes=str2num('[int32(2)]')  MultiplexTypes=str2num('[int32(1)]')  MultiplexValues=str2num('[double(0)]')  Factors=str2num('[double(1)]')  Offsets=str2num('[double(0)]')  Minimums=str2num('[double(0)]')  Maximums=str2num('[double(1)]')  Remote=off
      settings: DataFormat=CANdb specified signals
  CAN Transmit5 : canlib/CAN Transmit  BlockHandle=13267.0195  DeviceMenu=Vector Virtual 1 (Channel 1)  Device=Vector Virtual 1 (Channel 1)  ObjConstructor=canChannel('Vector', 'Virtual 1', 1)  EnablePeriodicTransmit=off  MessagePeriod=1.000
  Data Type Conversion1 : DataTypeConversion
  Rate Transition : RateTransition
  wires:
  Mode/1 -> Bus Selector3/1
  Data Type Conversion1/1 -> Rate Transition/1  "Mode"
  CAN Pack5/1 -> CAN Transmit5/1
  Bus Selector3/1 -> Data Type Conversion1/1  "<Mode>"
  Rate Transition/1 -> CAN Pack5/1

== system EcoSIM3_P2_C2/Powertrain/BAS Motor/Soft ECU/Algorithm/BAS_Stateflow/EEPROM Parameters ==
  note: Need to change this to reflect max speed of the BAS
  Bus Creator : BusCreator  Inputs=2
  Motor_MaxSpeed : Constant  Value=Plants.ICE.Mdl.Plant.red_line_w*Plants.Belt.GR
  POST_Fault : Constant  Value=0
  EEPROM param : Outport
  wires:
  Motor_MaxSpeed/1 -> Bus Creator/1  "Motor_MaxSpeed"
  Bus Creator/1 -> EEPROM param/1
  POST_Fault/1 -> Bus Creator/2  "POST_Fault"

== system EcoSIM3_P2_C2/Powertrain/BAS Motor/Soft ECU/Algorithm/BAS_Stateflow/Faults ==
  Bus Creator : BusCreator  Inputs=3
  Fault_U : Constant  Value=0
  Fault_V : Constant  Value=0
  Fault_W : Constant  Value=0
  Logical Operator : Logic  Operator=OR  Inputs=3  AllPortsSameDT=off  OutDataTypeStr=boolean
  MotorFault : Outport
  CAN : Outport  Port=2
  wires:
  Fault_V/1 -> Logical Operator/2, Bus Creator/2  "Fault_V"
  Bus Creator/1 -> CAN/1
  Fault_U/1 -> Logical Operator/3, Bus Creator/1  "Fault_U"
  Fault_W/1 -> Logical Operator/1, Bus Creator/3  "Fault_W"
  Logical Operator/1 -> MotorFault/1  "MotorFault"

== system EcoSIM3_P2_C2/Powertrain/BAS Motor/Soft ECU/Algorithm/BAS_Stateflow/Subsystem ==
  Speed_command_rpm : Inport
  Speed_feedback_rad_per_s : Inport  Port=2
  Gain1 : Gain  Gain=2*pi/60
  PID Controller : simulink/Continuous/PID Controller  Controller=PID  TimeDomain=Continuous-time  SampleTime=-1  IntegratorMethod=Forward Euler  FilterMethod=Forward Euler  Form=Parallel  P=2.0267926928279  I=0.12  D=-0.0833653881727756  N=24.31216044514  InitialConditionSource=internal  InitialConditionForIntegrator=0  InitialConditionForFilter=0  ExternalReset=none  LimitOutput=off  UpperSaturationLimit=inf  LowerSaturationLimit=-inf  LinearizeAsGain=on  AntiWindupMode=none  Kb=1  TrackingMode=off  Kt=1  PParamMin=[]  PParamMax=[]  IParamMin=[]  IParamMax=[]  DParamMin=[]  DParamMax=[]  NParamMin=[]  NParamMax=[]  KbParamMin=[]  KbParamMax=[]  KtParamMin=[]  KtParamMax=[]  POutMin=[]  POutMax=[]  IOutMin=[]  IOutMax=[]  DOutMin=[]  DOutMax=[]  NOutMin=[]  NOutMax=[]  KbOutMin=[]  KbOutMax=[]  KtOutMin=[]  KtOutMax=[]  IntegratorOutMin=[]  IntegratorOutMax=[]  FilterOutMin=[]  FilterOutMax=[]  SumOutMin=[]  SumOutMax=[]  SumI1OutMin=[]  SumI1OutMax=[]  SumI2OutMin=[]  SumI2OutMax=[]  SumI3OutMin=[]  SumI3OutMax=[]  SumDOutMin=[]  SumDOutMax=[]  SaturationOutMin=[]  SaturationOutMax=[]  IntegratorContinuousStateAttributes=''  IntegratorStateMustResolveToSignalObject=off  IntegratorRTWStateStorageClass=Auto  FilterContinuousStateAttributes=''  FilterStateMustResolveToSignalObject=off  FilterRTWStateStorageClass=Auto  DifferentiatorICPrevScaledInput=0  DifferentiatorOutMin=[]  DifferentiatorOutMax=[]  UseFilter=on
  Sum : Sum  Inputs=|+-
  "Torque_command_Nm " : Outport
  wires:
  Gain1/1 -> Sum/1
  Sum/1 -> PID Controller/1
  PID Controller/1 -> "Torque_command_Nm "/1
  Speed_feedback_rad_per_s/1 -> Sum/2
  Speed_command_rpm/1 -> Gain1/1

== system EcoSIM3_P2_C2/Powertrain/Electric Motor / Component Model/Plant/EM_Thermal_Model/EM_Over_Temp_Fault ==
  In1 : Inport
  Bus Selector : BusSelector  OutputSignals=Temp_deg_C,EM_OverTemp_Trigger
  Switch : Switch  Criteria=u2 > Threshold  Threshold=0.5
  Out1 : Outport
  wires:
  [EM_Over_temperature_Trigger] -> Bus Selector/1
  Bus Selector/1 -> Switch/1  "<Temp_deg_C>"
  Bus Selector/2 -> Switch/2  "<EM_OverTemp_Trigger>"
  Switch/1 -> Out1/1
  In1/1 -> Switch/3

== system EcoSIM3_P2_C2/Powertrain/Electric Motor / Component Model/Plant/EM_Thermal_Model/Heat Dissipated through coolant ==
  Coolant Out Temp : Inport
  Add1 : Sum  Inputs=+-
  Coolant Heat Capacity : Gain  Gain=3148
  Coolant Flow rate lit/min : Constant  Value=4
  Coolant Inlet Temp (K) : Constant  Value=293
  Product : Product
  Simulink-PS Converter2 : nesl_utility/Simulink-PS Converter  PhysicalDomain=network_engine_domain  SubClassName=ps_input  LeftPortType=input  RightPortType=output  PseudoPeriodic=off  Frequencies=[]  NoiseDistribution=none  NoiseParameters=[]  Unit=J/s  AffineConversion=off  InputFiltering=off  SimscapeFilterOrder=1  InputFilterTimeConstant=0.001  UdotUserProvided=1
  Subtract : Gain  Gain=-1
  per sec : Gain  Gain=1/60
  Coolant Heat Gain : PMIOPort  Port=1  Side=Right
  wires:
  Product/1 -> Subtract/1  "EM_Coolant_Heat_Reject_W"
  Coolant Heat Capacity/1 -> Product/2
  Add1/1 -> Product/1
  Coolant Inlet Temp (K)/1 -> Add1/2
  Subtract/1 -> Simulink-PS Converter2/1
  Coolant Out Temp/1 -> Add1/1
  per sec/1 -> Coolant Heat Capacity/1
  Coolant Flow rate lit/min/1 -> per sec/1
  connections:
  Simulink-PS Converter2/RConn1 -- Coolant Heat Gain/RConn1

== system EcoSIM3_P2_C2/Powertrain/Electric Motor / Component Model/Plant/EM_Thermal_Model/Temp Hotspot ==
  Add1 : Sum  Inputs=+-
  Constant3 : Constant  Value=273
  Ideal Temperature Sensor1 : fl_lib/Thermal/Thermal Sensors/Ideal Temperature Sensor
  PS-Simulink Converter1 : nesl_utility/PS-Simulink Converter  PhysicalDomain=network_engine_domain  SubClassName=ps_output  LeftPortType=input  RightPortType=output  PseudoPeriodic=off  Frequencies=[]  Unit=K  AffineConversion=off
  Thermal Reference5 : fl_lib/Thermal/Thermal Elements/Thermal Reference
  Conn1 : PMIOPort  Port=1  Side=Left
  Temp C : Outport
  wires:
  Constant3/1 -> Add1/2
  PS-Simulink Converter1/1 -> Add1/1
  Add1/1 -> Temp C/1
  connections:
  Ideal Temperature Sensor1/RConn2 -- PS-Simulink Converter1/LConn1
  Thermal Reference5/LConn1 -- Ideal Temperature Sensor1/RConn1
  Ideal Temperature Sensor1/LConn1 -- Conn1/RConn1

== system EcoSIM3_P2_C2/Powertrain/Electric Motor / Component Model/Plant/EM_Thermal_Model/Temp Motor ==
  Add : Sum  Inputs=+-
  Constant2 : Constant  Value=273
  Ideal Temperature Sensor : fl_lib/Thermal/Thermal Sensors/Ideal Temperature Sensor
  PS-Simulink Converter : nesl_utility/PS-Simulink Converter  PhysicalDomain=network_engine_domain  SubClassName=ps_output  LeftPortType=input  RightPortType=output  PseudoPeriodic=off  Frequencies=[]  Unit=K  AffineConversion=off
  Thermal Reference1 : fl_lib/Thermal/Thermal Elements/Thermal Reference
  Temp in : PMIOPort  Port=1  Side=Left
  Temp K : Outport
  Temp C : Outport  Port=2
  wires:
  PS-Simulink Converter/1 -> Temp K/1, Add/1
  Add/1 -> Temp C/1
  Constant2/1 -> Add/2
  connections:
  Ideal Temperature Sensor/RConn2 -- PS-Simulink Converter/LConn1
  Thermal Reference1/LConn1 -- Ideal Temperature Sensor/RConn1
  Temp in/RConn1 -- Ideal Temperature Sensor/LConn1

== system EcoSIM3_P2_C2/Powertrain/Electric Motor / Component Model/Sensors/Sensors/Sensor lag ==
  i : Inport
  1st Order LPF of 1ms in Discrete Form : DiscreteTransferFcn  Numerator=[0.6321]  Denominator=[1 -0.3679]
  o : Outport
  wires:
  i/1 -> 1st Order LPF of 1ms in Discrete Form/1
  1st Order LPF of 1ms in Discrete Form/1 -> o/1

== system EcoSIM3_P2_C2/Powertrain/Electric Motor / Component Model/Sensors/Sensors/Sensor lag1 ==
  i : Inport
  1st Order LPF of 1ms in Discrete Form : DiscreteTransferFcn  Numerator=[0.6321]  Denominator=[1 -0.3679]
  o : Outport
  wires:
  i/1 -> 1st Order LPF of 1ms in Discrete Form/1
  1st Order LPF of 1ms in Discrete Form/1 -> o/1

== system EcoSIM3_P2_C2/Powertrain/Electric Motor /Soft ECU/Algorithm/Normal Operation/EEPROM Parameters1 ==
  note: Key Switch Mode Always set to 0. Refer to RMS Hardware user manual
  Bus Creator : BusCreator  Inputs=3
  KeySwMode : Constant  Value=0
  Motor_MaxSpeed : Constant  Value=max(Plants.EM.Mdl.Plant.max_min_w)
  POST_Fault : Constant  Value=0
  EEPROM param : Outport
  wires:
  Motor_MaxSpeed/1 -> Bus Creator/1  "Motor_MaxSpeed"
  KeySwMode/1 -> Bus Creator/2  "KeySwMode"
  Bus Creator/1 -> EEPROM param/1
  POST_Fault/1 -> Bus Creator/3  "POST_Fault"

== system EcoSIM3_P2_C2/Powertrain/Electric Motor /Soft ECU/Algorithm/Startup_Shutdown/EEPROM Parameters ==
  note: Key Switch Mode Always set to 0. Refer to RMS Hardware user manual
  Bus Creator : BusCreator  Inputs=3
  KeySwMode : Constant  Value=0
  Motor_MaxSpeed : Constant  Value=max(Plants.EM.Mdl.Plant.max_min_w)
  POST_Fault : Constant  Value=0
  EEPROM param : Outport
  wires:
  Motor_MaxSpeed/1 -> Bus Creator/1  "Motor_MaxSpeed"
  KeySwMode/1 -> Bus Creator/2  "KeySwMode"
  Bus Creator/1 -> EEPROM param/1
  POST_Fault/1 -> Bus Creator/3  "POST_Fault"

== system EcoSIM3_P2_C2/Powertrain/Electric Motor /Soft ECU/Algorithm/Temperature Values Dummy/ESS_Over_Temp_Fault ==
  In1 : Inport
  Bus Selector1 : BusSelector  OutputSignals=Temp_deg_C,EM_Inverter_OverTemp_Trigger
  Switch : Switch  Criteria=u2 > Threshold  Threshold=0.5
  Out1 : Outport
  wires:
  In1/1 -> Switch/3
  Switch/1 -> Out1/1
  Bus Selector1/2 -> Switch/2  "<EM_Inverter_OverTemp_Trigger>"
  [EM_Inverter_Over_temperature_Trigger] -> Bus Selector1/1
  Bus Selector1/1 -> Switch/1  "<Temp_deg_C>"

== system EcoSIM3_P2_C2/Powertrain/Electrical Storage System/ ESS Model/Plant/Electrical Plant Model/Current Calculation (Per Cell) ==
  note: 3
  P_in [W] : Inport
  Batt_volt [V] : Inport  Port=2
  Battery capacity1 : Gain  Gain=1/(Plants.ESS.Mdl.Plant.EPM.Curr_Calc.P)
  Divide : Product  Inputs=*/
  Batt_Current [A] : Outport
  Cell_Current [A] : Outport  Port=2
  wires:
  P_in [W]/1 -> Divide/1
  Divide/1 -> Batt_Current [A]/1, Battery capacity1/1  "Batt_Current_A"
  Batt_volt [V]/1 -> Divide/2
  Battery capacity1/1 -> Cell_Current [A]/1  "Batt_Cell_Current_A]"

== system EcoSIM3_P2_C2/Powertrain/Electrical Storage System/ ESS Model/Plant/Electrical Plant Model/Heat Calculation ==
  note: 315
  Cell_Current [A] : Inport
  R_cell [Ohms] : Inport  Port=2
  Fcn : Fcn  Expr=u^2
  Heat input for pack : Gain  Gain=Plants.ESS.Mdl.Plant.EPM.Heat_Calc.N
  Product : Product
  Batt_Heat [W] : Outport
  wires:
  Fcn/1 -> Product/1
  R_cell [Ohms]/1 -> Product/2
  Product/1 -> Heat input for pack/1
  Heat input for pack/1 -> Batt_Heat [W]/1  "Batt_Heat_W"
  Cell_Current [A]/1 -> Fcn/1

== system EcoSIM3_P2_C2/Powertrain/Electrical Storage System/ ESS Model/Plant/Electrical Plant Model/OCV Estimation ==
  note: if I>0 --> DISCHARGE
  note: if I<0 --> CHARGE
  SOC [%] : Inport
  Cell_Current [A] : Inport  Port=2
  Charge : Subsystem
  Discharge : Subsystem
  Switch CHARGE OR DISCHARGE : Switch  Criteria=u2 > Threshold
  OCV [V] : Outport
  wires:
  Discharge/1(OCV [V]) -> Switch CHARGE OR DISCHARGE/1
  Charge/1(OCV [V]) -> Switch CHARGE OR DISCHARGE/3
  Cell_Current [A]/1 -> Switch CHARGE OR DISCHARGE/2
  Switch CHARGE OR DISCHARGE/1 -> OCV [V]/1  "Batt_Cell_OCV_V"
  SOC [%]/1 -> Discharge/1(SOC [%]), Charge/1(SOC [%])

== system EcoSIM3_P2_C2/Powertrain/Electrical Storage System/ ESS Model/Plant/Electrical Plant Model/Resistance Estimation (Per Cell)  ==
  note: if I>0 --> DISCHARGE
  note: if I<0 --> CHARGE
  Cell_Current [A] : Inport
  Cell_Temp [C] : Inport  Port=2
  SOC [%] : Inport  Port=3
  Charge : Subsystem
  Discharge : Subsystem
  Switch CHARGE OR DISCHARGE : Switch  Criteria=u2 > Threshold
  R_cell [Ohms] : Outport
  wires:
  Discharge/1(R_cell [Ohms]) -> Switch CHARGE OR DISCHARGE/1
  Charge/1(R_cell [Ohms]) -> Switch CHARGE OR DISCHARGE/3
  Cell_Current [A]/1 -> Switch CHARGE OR DISCHARGE/2
  Switch CHARGE OR DISCHARGE/1 -> R_cell [Ohms]/1  "Batt_Cell_Resistance_Ohms"
  Cell_Temp [C]/1 -> Charge/1(Temp [C]), Discharge/1(Temp [C])
  SOC [%]/1 -> Discharge/2(SOC [%]), Charge/2(SOC [%])

== system EcoSIM3_P2_C2/Powertrain/Electrical Storage System/ ESS Model/Plant/Electrical Plant Model/SOC Estimation (Per Cell) ==
  note: 1/Gain2
  note: Gain2
  note: (19.6*3600*1000)/100
  note: -1 What is this?
  P_in [W] : Inport
  A.h to A.sec1 : Gain  Gain=1/Plants.ESS.Mdl.Plant.EPM.SOC_Est.Gain2
  Bus Selector : BusSelector  OutputSignals=Init_SOC_percent
  Gain1 : Gain  Gain=Plants.ESS.Mdl.Plant.EPM.SOC_Est.Gain1
  Integrator Limited : Integrator  InitialConditionSource=external  InitialCondition=19.6*3600*1000  LimitOutput=on  UpperSaturationLimit=19.6*3600*1000  LowerSaturationLimit=0
  SOC : Gain  Gain=Plants.ESS.Mdl.Plant.EPM.SOC_Est.Gain2
  SOC [%] : Outport
  wires:
  Integrator Limited/1 -> A.h to A.sec1/1
  Gain1/1 -> Integrator Limited/1
  P_in [W]/1 -> Gain1/1
  A.h to A.sec1/1 -> SOC [%]/1  "Batt_SOC_percent"
  SOC/1 -> Integrator Limited/2
  [Simulation_Parameters] -> Bus Selector/1
  Bus Selector/1 -> SOC/1  "<Init_SOC_percent>"

== system EcoSIM3_P2_C2/Powertrain/Electrical Storage System/ ESS Model/Plant/Electrical Plant Model/Terminal Voltage Calculation ==
  note: 105
  R_cell [Ohms] : Inport
  OCV [V] : Inport  Port=2
  Cell_Current [A] : Inport  Port=3
  Add : Sum  Inputs=+-
  Pack voltage : Gain  Gain=Plants.ESS.Mdl.Plant.EPM.Term_V_calc.S
  Product1 : Product
  Batt_Volt [V] : Outport
  wires:
  Product1/1 -> Add/2
  Add/1 -> Pack voltage/1
  OCV [V]/1 -> Add/1
  Cell_Current [A]/1 -> Product1/1
  R_cell [Ohms]/1 -> Product1/2
  Pack voltage/1 -> Batt_Volt [V]/1  "Batt_Voltage_V"

== system EcoSIM3_P2_C2/Powertrain/Electrical Storage System/ ESS Model/Plant/Power Calculation/Avg Power Calculation ==
  note: EM+BAS+Accessories
  Input_Crnt [A] : Inport
  Batt_volt_1 [V] : Inport  Port=2
  Component_Power_Watts : Inport  Port=3
  " " : Sum  SaturateOnIntegerOverflow=on  InputSameDT=on  OutDataTypeStr=Inherit: Same as first input
  Divide1 : Product  Inputs=**
  P_in [W] : Outport
  wires:
  Input_Crnt [A]/1 -> Divide1/1
  Batt_volt_1 [V]/1 -> Divide1/2
  Divide1/1 -> " "/1
  " "/1 -> P_in [W]/1  "Batt_P_In_W"
  Component_Power_Watts/1 -> " "/2

== system EcoSIM3_P2_C2/Powertrain/Electrical Storage System/ ESS Model/Plant/Thermal Model/EM_Over_Temp_Fault ==
  In1 : Inport
  Bus Selector : BusSelector  OutputSignals=Temp_deg_C,ESS_OverTemp_Trigger
  Switch : Switch  Criteria=u2 > Threshold  Threshold=0.5
  Out1 : Outport
  wires:
  [ESS_Over_temperature_Trigger] -> Bus Selector/1
  Bus Selector/1 -> Switch/1  "<Temp_deg_C>"
  Bus Selector/2 -> Switch/2  "<ESS_OverTemp_Trigger>"
  Switch/1 -> Out1/1
  In1/1 -> Switch/3

== system EcoSIM3_P2_C2/Powertrain/Soft_ECUs_IO/VNT Kvaser/CANTx/EM/M160_Temperature_Set_1 ==
  EM : Inport
  Bus Selector5 : BusSelector  OutputSignals=M160_Temperature_Set_1.Module_A,M160_Temperature_Set_1.Module_B,M160_Temperature_Set_1.Module_C,M160_Temperature_Set_1.Gate_Driver_Board
  CAN Pack3 : canmsglib/CAN Pack  CANdbFile=C:\Users\EcoCAR_HIL\Documents\Khanna\EcoSIM3_P1_0_PHEV_TCU\Final_DBC\20150828 RMS PM CAN DB.dbc  MsgList=M160_Temperature_Set_1  MsgName=M160_Temperature_Set_1  MsgIDType=Standard (11-bit identifier)  MsgIdentifier=160  MsgLength=8  SignalInfo=D1_Module_A$0$16$1$1$1$0$1.000000e-01$0$-3.276800e+03$3.276700e+03$#D2_Module_B$16$16$1$1$1$0$1.000000e-01$0$-3.276800e+03$3.276700e+03$#D3_Module_C$32$16$1$1$1$0$1.000000e-01$0$-3.276800e+03$3.276700e+03$#D4_Gate_Driver_Board$48$16$1$1$1$0$1.000000e-01$0$-3.276800e+03$3.276700e+03$#  NSignals=4  StartBits=str2num('[int32(0);int32(16);int32(32);int32(48)]')  SignalSizes=str2num('[int32(16);int32(16);int32(16);int32(16)]')  ByteOrders=str2num('[int32(1);int32(1);int32(1);int32(1)]')  DataTypes=str2num('[int32(1);int32(1);int32(1);int32(1)]')  MultiplexTypes=str2num('[int32(1);int32(1);int32(1);int32(1)]')  MultiplexValues=str2num('[double(0);double(0);double(0);double(0)]')  Factors=str2num('[double(1.000000e-01);double(1.000000e-01);double(1.000000e-01);double(1.000000e-01)]')  Offsets=str2num('[double(0);double(0);double(0);double(0)]')  Minimums=str2num('[double(-3.276800e+03);double(-3.276800e+03);double(-3.276800e+03);double(-3.276800e+03)]')  Maximums=str2num('[double(3.276700e+03);double(3.276700e+03);double(3.276700e+03);double(3.276700e+03)]')  Remote=off
      settings: DataFormat=CANdb specified signals
  CAN Transmit1 : canlib/CAN Transmit  BlockHandle=2890.0023  DeviceMenu=Kvaser Virtual 1 (Channel 2)  Device=Kvaser Virtual 1 (Channel 2)  ObjConstructor=canChannel('Kvaser', 'Virtual 1', 2)  EnablePeriodicTransmit=off  MessagePeriod=1.000
  Rate Transition{,1..3} (4 alike) : RateTransition
  wires:
  Bus Selector5/2 -> Rate Transition3/1  "<Module_B>"
  Bus Selector5/4 -> Rate Transition1/1  "<Gate_Driver_Board>"
  Bus Selector5/1 -> Rate Transition/1  "<Module_A>"
  Bus Selector5/3 -> Rate Transition2/1  "<Module_C>"
  EM/1 -> Bus Selector5/1
  Rate Transition/1 -> CAN Pack3/1
  Rate Transition1/1 -> CAN Pack3/4
  Rate Transition2/1 -> CAN Pack3/3
  Rate Transition3/1 -> CAN Pack3/2
  CAN Pack3/1 -> CAN Transmit1/1
